simulink model "AeroPlantMIAC"  (R2020b)
settings: Solver=ode45  StartTime=0.0  StopTime=50.0  RelTol=1e-3  EnableMultiTasking=on
model workspace: external: MATLAB File D:\Documents\Masters\Adaptive Control\Lab\Ex4MatlabFiles\init_miac.m (data not in the file)
values from neighbouring files (symbols this model uses):
  sigma2e = 0.01    [init_miac.m]    (also in init_mrac.m = 0; init_mraclb.m = 0)
  Ta = 0.04    [init_adrc.m]    (also in init_miac.m = 0.05)
  Tc = 0.1    [init_adrc.m]    (also in init_miac.m = 0.001; init_mrac.m; init_mraclb.m)
  TF = 1.5*Ta    (= 0.075)    [init_miac.m]
  wr = 0.25    [init_miac.m]    (also in init_mrac.m; init_mraclb.m = 0.15)
  Yr = 0.15    [init_miac.m]
libraries: simulink x1
settings Model: ModifiedComment=Melkamu A -- Sun May 12 18:32:48 2024 -- Version 1.21  ModifiedHistory=Melkamu A -- Sun May 12 18:32:48 2024 -- Version 1.21  OrderedModelArguments=off  Creator=Melkamu A  LastModifiedBy=Melkamu A
settings DataIOCC: LimitDataPoints=on  SaveFinalState=on  SaveOperatingPoint=on  SaveFormat=Array  SignalLoggingSaveFormat=ModelDataLogs  SaveState=on  SignalLogging=off  ReturnWorkspaceOutputs=off
settings OptimizationCC: InitFltsAndDblsToZero=on  LifeSpan=inf
settings DebuggingCC: SaveWithParameterizedLinksMsg=none  UnderspecifiedInitializationDetection=Classic  MergeDetectMultiDrivingBlocksExec=none  SignalResolutionControl=TryResolveAllWithWarning  SolverPrmCheckMsg=warning  MultiTaskDSMMsg=warning  MultiTaskCondExecSysMsg=none  FcnCallInpInsideContextMsg=warning  SFUnexpectedBacktrackingDiag=warning  SFNoUnconditionalDefaultTransitionDiag=warning  SFExecutionAtInitializationDiag=none  ArithmeticOperatorsInVariantConditions=warning
settings HardwareCC: ProdBitPerPointer=32  ProdBitPerSizeT=32  ProdBitPerPtrDiffT=32  ProdLargestAtomicFloat=None  ProdIntDivRoundTo=Undefined  ProdEndianess=Unspecified  ProdWordSize=32  ProdHWDeviceType=32-bit Generic
settings ModelReferenceCC: PropagateSignalLabelsOutOfModel=off
settings CodeAppCC: StateflowObjectComments=on
settings GRTTargetCC: TargetFcnLib=ansi_tfl_tmw.mat  TargetLangStandard=C89/C90 (ANSI)  CombineOutputUpdateFcns=off  GRTInterface=on
settings ConfigComp: CovMetricSettings=dw  CovSaveCumulativeToWorkspaceVar=on  CovSaveSingleToWorkspaceVar=on

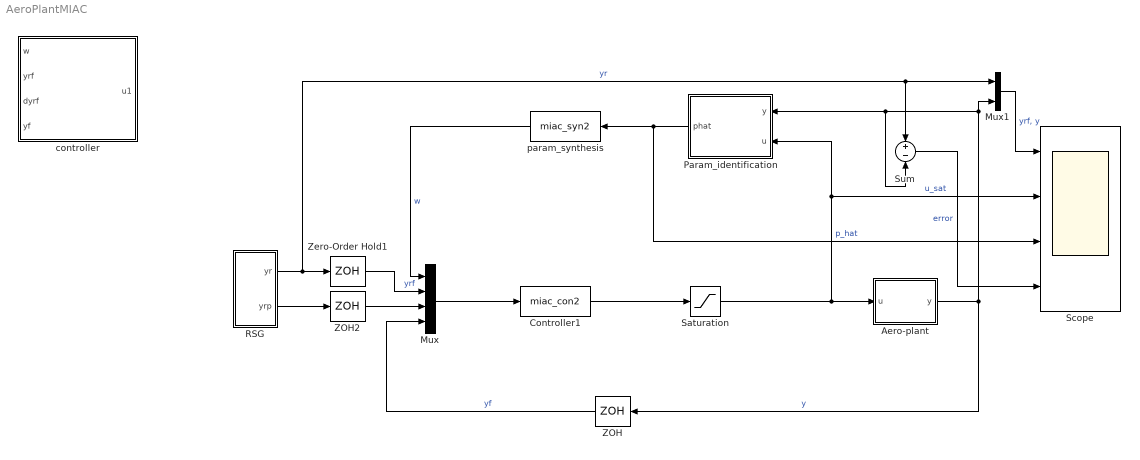
== system AeroPlantMIAC ==
  Aero-plant : Subsystem
  Controller1 : MATLABFcn  MATLABFcn=miac_con2  OutputDimensions=1
  Mux : Mux  Inputs=[3 1 1 1]
  Mux1 : Mux  Inputs=2
  Param_identification : Subsystem
  RSG : Subsystem
  Saturation : Saturate  UpperLimit=pi  LowerLimit=-pi
  Scope : Scope  NumInputPorts=4
  Sum : Sum  Inputs=+-
  ZOH : ZeroOrderHold  SampleTime=Tc
  ZOH2 : ZeroOrderHold  SampleTime=Tc
  Zero-Order Hold1 : ZeroOrderHold  SampleTime=Tc
  controller : Subsystem
  param_synthesis : MATLABFcn  MATLABFcn=miac_syn2
  wires:
  param_synthesis/1 -> Mux/1  "w"
  Aero-plant/1(y) -> Param_identification/1(y), Sum/2, Mux1/2, ZOH/1  "y"
  RSG/2(yrp) -> ZOH2/1
  RSG/1(yr) -> Sum/1, Mux1/1, Zero-Order Hold1/1  "yr"
  ZOH/1 -> Mux/4  "yf"
  ZOH2/1 -> Mux/3
  Zero-Order Hold1/1 -> Mux/2  "yrf"
  Mux/1 -> Controller1/1
  Param_identification/1(phat) -> Scope/3, param_synthesis/1  "p_hat"
  Mux1/1 -> Scope/1  "yrf, y"
  Sum/1 -> Scope/4  "error"
  Controller1/1 -> Saturation/1
  Saturation/1 -> Param_identification/2(u), Scope/2, Aero-plant/1(u)  "u_sat"

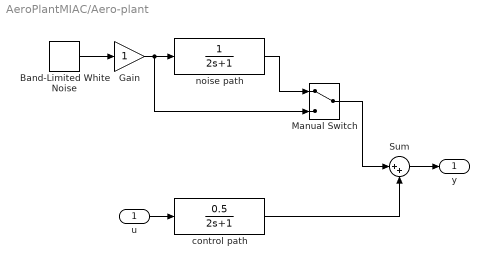
== system AeroPlantMIAC/Aero-plant ==
  u : Inport
  Band-Limited White Noise : simulink/Sources/Band-Limited White Noise  Cov=[sigma2e*Tc]  Ts=Tc  seed=[23341]
  Gain : Gain
  Manual Switch : ManualSwitch
  Sum : Sum  Inputs=|++
  control path : TransferFcn  Numerator=[0.5]  Denominator=[2 1]
  noise path : TransferFcn  Denominator=[2 1]
  y : Outport
  wires:
  Band-Limited White Noise/1 -> Gain/1
  Gain/1 -> Manual Switch/2, noise path/1
  control path/1 -> Sum/2
  u/1 -> control path/1
  noise path/1 -> Manual Switch/1
  Manual Switch/1 -> Sum/1
  Sum/1 -> y/1

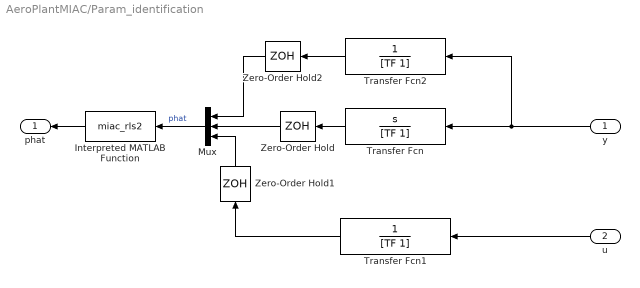
== system AeroPlantMIAC/Param_identification ==
  y : Inport
  u : Inport  Port=2
  Interpreted MATLAB Function : MATLABFcn  MATLABFcn=miac_rls2  OutputDimensions=2
  Mux : Mux  Inputs=3
  Transfer Fcn : TransferFcn  Numerator=[1 0]  Denominator=[TF 1]
  Transfer Fcn1 : TransferFcn  Denominator=[TF 1]
  Transfer Fcn2 : TransferFcn  Denominator=[TF 1]
  Zero-Order Hold : ZeroOrderHold  SampleTime=Ta
  Zero-Order Hold1 : ZeroOrderHold  SampleTime=Ta
  Zero-Order Hold2 : ZeroOrderHold  SampleTime=Ta
  phat : Outport
  wires:
  Mux/1 -> Interpreted MATLAB Function/1  "phat"
  Transfer Fcn1/1 -> Zero-Order Hold1/1
  Zero-Order Hold/1 -> Mux/2
  y/1 -> Transfer Fcn2/1, Transfer Fcn/1
  Zero-Order Hold1/1 -> Mux/3
  Zero-Order Hold2/1 -> Mux/1
  Transfer Fcn/1 -> Zero-Order Hold/1
  Transfer Fcn2/1 -> Zero-Order Hold2/1
  u/1 -> Transfer Fcn1/1
  Interpreted MATLAB Function/1 -> phat/1

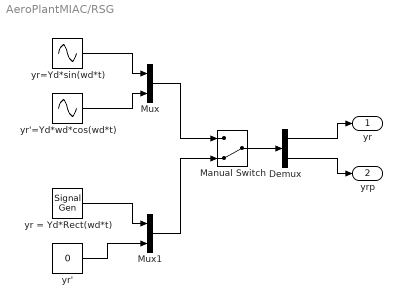
== system AeroPlantMIAC/RSG ==
  Demux : Demux  Outputs=2
  Manual Switch : ManualSwitch  CurrentSetting=0
  Mux : Mux  Inputs=2
  Mux1 : Mux  Inputs=2
  yr = Yd*Rect(wd*t) : SignalGenerator  WaveForm=square  Amplitude=Yr  Frequency=wr  Units=rad/sec
  yr' : Constant  Value=0
  yr'=Yd*wd*cos(wd*t) : Sin  Amplitude=Yr*wr  Frequency=wr  Phase=pi/2  SampleTime=0
  yr=Yd*sin(wd*t) : Sin  Amplitude=Yr  Frequency=wr  SampleTime=0
  yr : Outport
  yrp : Outport  Port=2
  wires:
  yr=Yd*sin(wd*t)/1 -> Mux/1
  yr'=Yd*wd*cos(wd*t)/1 -> Mux/2
  yr = Yd*Rect(wd*t)/1 -> Mux1/1
  yr'/1 -> Mux1/2
  Mux/1 -> Manual Switch/1
  Mux1/1 -> Manual Switch/2
  Manual Switch/1 -> Demux/1
  Demux/1 -> yr/1
  Demux/2 -> yrp/1

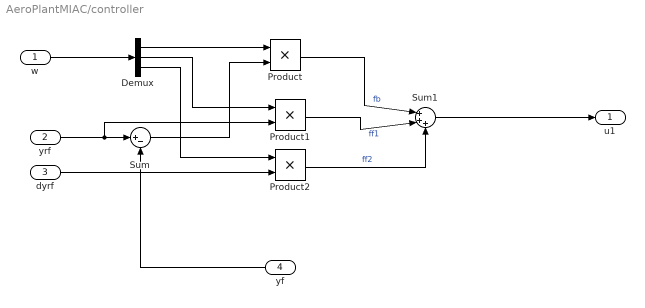
== system AeroPlantMIAC/controller ==
  w : Inport
  yrf : Inport  Port=2
  dyrf : Inport  Port=3
  yf : Inport  Port=4
  Demux : Demux  Outputs=3
  Product : Product
  Product1 : Product
  Product2 : Product
  Sum : Sum  Inputs=|+-
  Sum1 : Sum  Inputs=|+++
  u1 : Outport
  wires:
  yrf/1 -> Product1/2, Sum/1
  Demux/3 -> Product2/1
  Product/1 -> Sum1/1  "fb"
  Demux/1 -> Product/1
  Sum/1 -> Product/2
  w/1 -> Demux/1
  Demux/2 -> Product1/1
  Product1/1 -> Sum1/2  "ff1"
  Product2/1 -> Sum1/3  "ff2"
  dyrf/1 -> Product2/2
  yf/1 -> Sum/2
  Sum1/1 -> u1/1
